simulink model "simple_simulink_state_space_simulation_with_initial_state"  (R2021a)
settings: Solver=VariableStepAuto  StartTime=0.0  StopTime=10.0  RelTol=1e-3
settings Model: Creator=User  LastModifiedBy=User

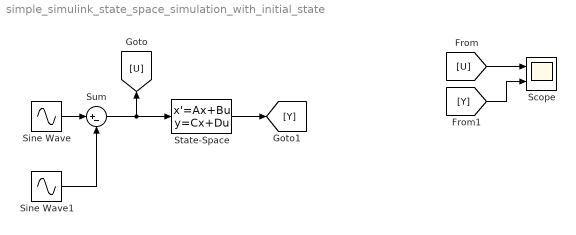
== system simple_simulink_state_space_simulation_with_initial_state ==
  Scope : Scope  NumInputPorts=2
  Sine Wave : Sin  Amplitude=30  Frequency=2  SampleTime=0
  Sine Wave1 : Sin  Amplitude=10  Frequency=4  Phase=pi/2  SampleTime=0
  State-Space : StateSpace  A=[0 1; -50 -0.1]  B=[0; 10]  C=[1 0]  D=0  InitialCondition=0
  Sum : Sum  Inputs=|+-
  wires:
  Sine Wave/1 -> Sum/1
  Sine Wave1/1 -> Sum/2
  Sum/1 -> [U], State-Space/1
  [U] -> Scope/1
  State-Space/1 -> [Y]
  [Y] -> Scope/2
